simulink model "STOICAL_example_1_Step01c_DefineSignals"  (R2014b)
settings: Solver=ode4  StartTime=0.0  StopTime=1  FixedStep=50E-6  RelTol=1e-3
settings Model: Creator=Wippenbeck  LastModifiedBy=Wippenbeck

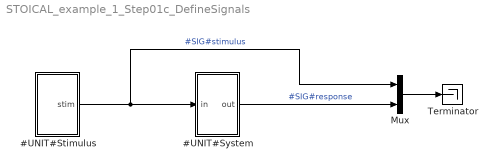
== system STOICAL_example_1_Step01c_DefineSignals ==
  #UNIT#Stimulus : Subsystem
  #UNIT#System : Subsystem
  Mux : Mux  Inputs=2
  Terminator : Terminator
  wires:
  Mux/1 -> Terminator/1
  #UNIT#Stimulus/1(stim) -> #UNIT#System/1(in), Mux/1  "#SIG#stimulus"
  #UNIT#System/1(out) -> Mux/2  "#SIG#response"

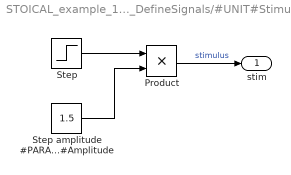
== system STOICAL_example_1_Step01c_DefineSignals/#UNIT#Stimulus ==
  Product : Product
  Step : Step  Time=0.1  SampleTime=0
  Step amplitude #PARAM#Amplitude : Constant  Value=1.5
  stim : Outport
  wires:
  Step amplitude #PARAM#Amplitude/1 -> Product/2
  Product/1 -> stim/1  "stimulus"
  Step/1 -> Product/1

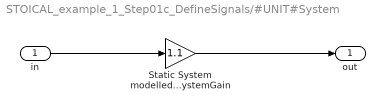
== system STOICAL_example_1_Step01c_DefineSignals/#UNIT#System ==
  in : Inport
  Static System modelled by gain block #PARAM#SystemGain : Gain  Gain=1.1
  out : Outport
  wires:
  Static System modelled by gain block #PARAM#SystemGain/1 -> out/1
  in/1 -> Static System modelled by gain block #PARAM#SystemGain/1
